simulink model "QAWUP"  (Simulink 3.00)
settings: Solver=ode45  SolverMode=SingleTasking  StartTime=0.0  StopTime=20  MaxStep=0.010  RelTol=1e-3  AbsTol=1e-3
undefined symbols (not defined in the file or in its folder): dqi, nqi, qi, sat
settings Model: TimeSaveName=t  SaveOutput=off

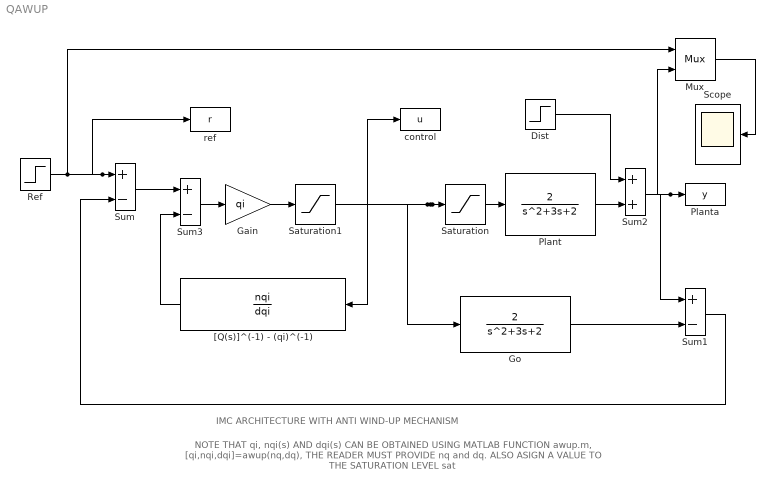
== system QAWUP ==
  note: IMC ARCHITECTURE WITH ANTI WIND-UP MECHANISM
  note: NOTE THAT qi, nqi(s) AND dqi(s) CAN BE OBTAINED USING MATLAB FUNCTION awup.m,
      | [qi,nqi,dqi]=awup(nq,dq), THE READER MUST PROVIDE nq and dq. ALSO ASIGN A VALUE TO
      | THE SATURATION LEVEL sat
  Dist : Step  Time=10  Before=0  After=-1  SampleTime=0
  Gain : Gain  Gain=qi  SaturateOnIntegerOverflow=on
  Go : TransferFcn  Numerator=2  Denominator=[1 3 2]
  Mux : Mux  Inputs=2
      settings: DisplayOption=none
  Plant : TransferFcn  Numerator=2  Denominator=[1 3 2]
  Planta : ToWorkspace  VariableName=y  SampleTime=0  SaveFormat=Matrix
      settings: Buffer=6000
  Ref : Step  Time=1  Before=0  After=1  SampleTime=0
  Saturation : Saturate  UpperLimit=sat  LowerLimit=-sat
  Saturation1 : Saturate  UpperLimit=sat  LowerLimit=-sat
  Scope : Scope
      settings: TickLabels=on  TimeRange=20.000000  YMin=-1.2  YMax=1.2  SaveToWorkspace=off  SaveName=ScopeData  DataFormat=Matrix
  Sum : Sum  Inputs=+-  SaturateOnIntegerOverflow=on
  Sum1 : Sum  Inputs=+-  SaturateOnIntegerOverflow=on
  Sum2 : Sum  Inputs=++  SaturateOnIntegerOverflow=on
  Sum3 : Sum  Inputs=+-  SaturateOnIntegerOverflow=on
  "[Q(s)]^(-1) - (qi)^(-1)" : TransferFcn  Orientation=left  Numerator=nqi  Denominator=dqi  mask{nqi=nqi, dqi=dqi}
      mask prompts: nqi "numerator (nqi)"; dqi "denominator (dqi)"
      mask help: [Q(s)]^(-1) - (qi)^(-1)
      mask Display: disp('[Q(s)]^(-1) - (qi)^(-1)')
  control : ToWorkspace  VariableName=u  SampleTime=0  SaveFormat=Matrix
      settings: Buffer=6000
  ref : ToWorkspace  VariableName=r  SampleTime=0  SaveFormat=Matrix
      settings: Buffer=6000
  wires:
  Go/1 -> Sum1/2
  Sum1/1 -> Sum/2
  Plant/1 -> Sum2/2
  Dist/1 -> Sum2/1
  Saturation/1 -> Plant/1
  Sum3/1 -> Gain/1
  Sum/1 -> Sum3/1
  "[Q(s)]^(-1) - (qi)^(-1)"/1 -> Sum3/2
  Saturation1/1 -> "[Q(s)]^(-1) - (qi)^(-1)"/1, Saturation/1, Go/1, control/1
  Gain/1 -> Saturation1/1
  Mux/1 -> Scope/1
  Ref/1 -> Mux/1, Sum/1, ref/1
  Sum2/1 -> Mux/2, Sum1/1, Planta/1
